simulink model "0"  (R2019a)
settings: Solver=VariableStepAuto  StartTime=0.0  StopTime=10.0  RelTol=1e-3
values from neighbouring files (symbols this model uses):
  C = 1    [value.m]
  L = 1    [value.m]
  R = 1    [value.m]
settings Model: Creator=TakumiShiota  LastModifiedBy=TakumiShiota

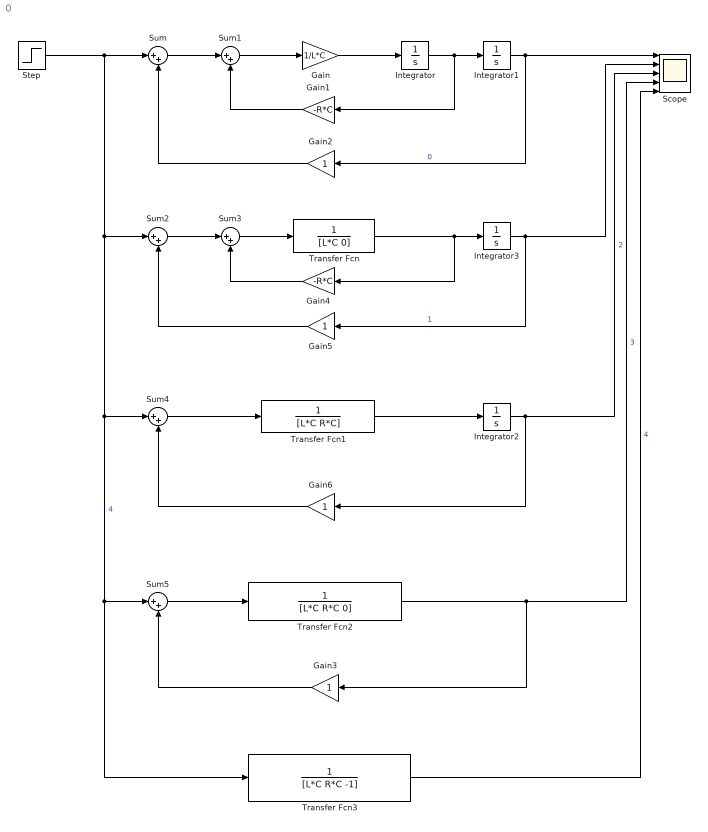
== system 0 ==
  Gain : Gain  Gain=1/L*C
  Gain1 : Gain  Gain=-R*C
  Gain{2..3,5..6} (4 alike) : Gain
  Gain4 : Gain  Gain=-R*C
  Integrator{,1..3} (4 alike) : Integrator
  Scope : Scope  NumInputPorts=5
  Step : Step  SampleTime=0
  Sum{,1..5} (6 alike) : Sum  Inputs=|++
  Transfer Fcn : TransferFcn  Denominator=[L*C 0]
  Transfer Fcn1 : TransferFcn  Denominator=[L*C R*C]
  Transfer Fcn2 : TransferFcn  Denominator=[L*C R*C 0]
  Transfer Fcn3 : TransferFcn  Denominator=[L*C R*C -1]
  wires:
  Integrator/1 -> Gain1/1, Integrator1/1
  Sum1/1 -> Gain/1
  Gain/1 -> Integrator/1
  Gain1/1 -> Sum1/2
  Sum/1 -> Sum1/1
  Step/1 -> Transfer Fcn3/1, Sum5/1, Sum4/1, Sum2/1, Sum/1  "4"
  Integrator1/1 -> Gain2/1, Scope/1  "0"
  Gain2/1 -> Sum/2
  Gain5/1 -> Sum2/2
  Integrator3/1 -> Scope/2, Gain5/1  "1"
  Transfer Fcn/1 -> Integrator3/1, Gain4/1
  Gain4/1 -> Sum3/2
  Sum2/1 -> Sum3/1
  Sum3/1 -> Transfer Fcn/1
  Sum4/1 -> Transfer Fcn1/1
  Transfer Fcn1/1 -> Integrator2/1
  Gain6/1 -> Sum4/2
  Integrator2/1 -> Gain6/1, Scope/3  "2"
  Gain3/1 -> Sum5/2
  Transfer Fcn2/1 -> Gain3/1, Scope/4  "3"
  Sum5/1 -> Transfer Fcn2/1
  Transfer Fcn3/1 -> Scope/5  "4"
